simulink model "prac6_sist_electricos_simulink"  (R2025a)
settings: Solver=ode45  StartTime=0.0  StopTime=0.002  RelTol=1e-3
InitFcn:
  | R=10;
  | L=0.002;
  | C=10e-6;
  | U_in = 32;
settings Model: Creator=USER  LastModifiedBy=USER

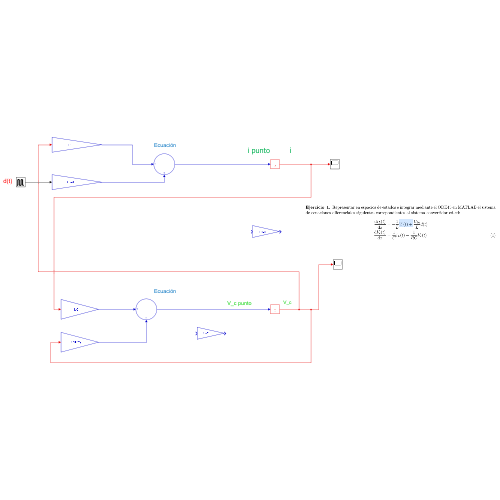
[thumbnail: Simulink's stored preview of the top-level diagram]
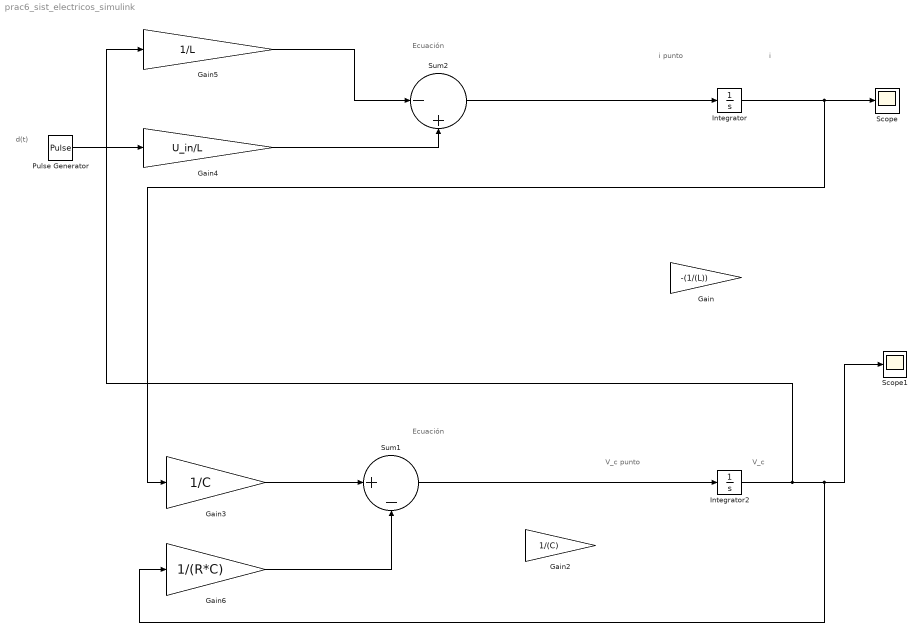
== system prac6_sist_electricos_simulink ==
  note: i
  note: i punto
  note: Ecuación
  note: Ecuación
  note: V_c punto
  note: d(t)
  note: V_c
  Gain : Gain  Gain=-(1/(L))
  Gain2 : Gain  Gain=1/(C)
  Gain3 : Gain  Gain=1/C
  Gain4 : Gain  Gain=U_in/L
  Gain5 : Gain  Gain=1/L
  Gain6 : Gain  Gain=1/(R*C)
  Integrator : Integrator
  Integrator2 : Integrator
  Pulse Generator : DiscretePulseGenerator  PulseType=Time based  Period=1/(100e3)  PulseWidth=40
  Scope : Scope
      settings: ActiveDisplayYMinimum=-0.17312047082165338  ActiveDisplayYMaximum=1.5580842373948807
  Scope1 : Scope
      settings: ActiveDisplayYMinimum=-1.6690763206549943  ActiveDisplayYMaximum=15.021686885894953
  Sum1 : Sum  Inputs=|+-
  Sum2 : Sum  Inputs=|-+
  wires:
  Gain3/1 -> Sum1/1
  Integrator/1 -> Scope/1, Gain3/1
  Integrator2/1 -> Gain5/1, Scope1/1, Gain6/1
  Gain6/1 -> Sum1/2
  Pulse Generator/1 -> Gain4/1
  Gain5/1 -> Sum2/1
  Gain4/1 -> Sum2/2
  Sum1/1 -> Integrator2/1
  Sum2/1 -> Integrator/1
